simulink model "sampleModel7288_pp_1_1"  (R2018a)
settings: Solver=VariableStepAuto  StartTime=0.0  StopTime=10.0  RelTol=1e-3
undefined symbols (not defined in the file): DiscIntNeverNeededParam, sigbuilder_block
libraries: simulink x497
(part 10 of 10)

== system sampleModel7288_pp_1_1/cfblk310/cfblk17 ==
  cfblk1 : Inport
  cfblk10 : Inport  Port=2
  Action Port : ActionPort  ActionType=else
  cfblk13 : Delay
  cfblk14 : Delay
  cfblk3 : Delay  ShowEnablePort=on
      settings: InputPortMap=u0,e6
  cfblk4 : Delay
  cfblk5 : Delay  ShowEnablePort=on
      settings: InputPortMap=u0,e6
  cfblk6 : DiscreteTransferFcn
  cfblk7 : DiscreteIntegrator  SampleTime=-1  OutDataTypeStr=double  ICPrevOutput=DiscIntNeverNeededParam  ICPrevScaledInput=DiscIntNeverNeededParam
  cfblk8 : simulink/Continuous/PID Controller (2DOF)  Controller=PID  TimeDomain=Discrete-time  SampleTime=-1  IntegratorMethod=Forward Euler  FilterMethod=Forward Euler  Form=Parallel  UseFilter=on  ControllerParametersSource=internal  P=1  I=1  D=0  N=100  b=1  c=1  InitialConditionSource=internal  InitialConditionForIntegrator=0  InitialConditionForFilter=0  ExternalReset=none  LimitOutput=off  UpperSaturationLimit=inf  LowerSaturationLimit=-inf  LinearizeAsGain=off  AntiWindupMode=none  Kb=1  TrackingMode=off  Kt=1  PParamMin=[]  PParamMax=[]  IParamMin=[]  IParamMax=[]  DParamMin=[]  DParamMax=[]  NParamMin=[]  NParamMax=[]  bParamMin=[]  bParamMax=[]  cParamMin=[]  cParamMax=[]  KbParamMin=[]  KbParamMax=[]  KtParamMin=[]  KtParamMax=[]  POutMin=[]  POutMax=[]  IOutMin=[]  IOutMax=[]  DOutMin=[]  DOutMax=[]  NOutMin=[]  NOutMax=[]  bOutMin=[]  bOutMax=[]  cOutMin=[]  cOutMax=[]  KbOutMin=[]  KbOutMax=[]  KtOutMin=[]  KtOutMax=[]  IntegratorOutMin=[]  IntegratorOutMax=[]  FilterOutMin=[]  FilterOutMax=[]  SumOutMin=[]  SumOutMax=[]  Sum1OutMin=[]  Sum1OutMax=[]  Sum2OutMin=[]  Sum2OutMax=[]  Sum3OutMin=[]  Sum3OutMax=[]  SumI1OutMin=[]  SumI1OutMax=[]  SumI2OutMin=[]  SumI2OutMax=[]  SumI3OutMin=[]  SumI3OutMax=[]  SumDOutMin=[]  SumDOutMax=[]  SaturationOutMin=[]  SaturationOutMax=[]  IntegratorContinuousStateAttributes=''  IntegratorStateMustResolveToSignalObject=off  IntegratorRTWStateStorageClass=Auto  FilterContinuousStateAttributes=''  FilterStateMustResolveToSignalObject=off  FilterRTWStateStorageClass=Auto  DifferentiatorICPrevScaledInput=0  DifferentiatorOutMin=[]  DifferentiatorOutMax=[]  FilterDiffOutCoefMin=[]  FilterDiffOutCoefMax=[]  SumDenOutMin=[]  SumDenOutMax=[]  SumNumOutMin=[]  SumNumOutMax=[]  ReciprocalOutMin=[]  ReciprocalOutMax=[]  DivideOutMin=[]  DivideOutMax=[]  TunerSelectOption=Transfer Function Based (PID Tuner App)
  cfblk9 : Delay  DelayLengthSource=Input port
      settings: InputPortMap=u0,p1
  cyemi_{1470..1482} (13 alike) : DataTypeConversion  OutDataTypeStr=double
  cfblk2 : Outport
  cfblk11 : Outport  Port=2
  cfblk12 : Outport  Port=3
  wires:
  cfblk9/1 -> cfblk12/1, cfblk11/1, cyemi_1476/1, cyemi_1479/1
  cfblk5/1 -> cfblk2/1, cyemi_1470/1, cyemi_1471/1
  cyemi_1470/1 -> cfblk13/1
  cyemi_1471/1 -> cfblk14/1
  cyemi_1472/1 -> cfblk3/1
  cfblk6/1 -> cyemi_1472/1
  cyemi_1473/1 -> cfblk3/2
  cfblk1/1 -> cyemi_1473/1
  cyemi_1474/1 -> cfblk4/1
  cfblk3/1 -> cyemi_1474/1
  cyemi_1475/1 -> cfblk5/1
  cfblk8/1 -> cyemi_1475/1
  cyemi_1476/1 -> cfblk5/2
  cyemi_1477/1 -> cfblk6/1
  cfblk10/1 -> cyemi_1477/1
  cyemi_1478/1 -> cfblk7/1
  cfblk4/1 -> cyemi_1478/1
  cyemi_1479/1 -> cfblk8/1
  cyemi_1480/1 -> cfblk8/2
  cfblk14/1 -> cyemi_1480/1
  cyemi_1481/1 -> cfblk9/1
  cfblk13/1 -> cyemi_1481/1
  cyemi_1482/1 -> cfblk9/2
  cfblk7/1 -> cyemi_1482/1

== system sampleModel7288_pp_1_1/cfblk311/cfblk18 ==
  cfblk1 : Inport
  cfblk13 : Inport  Port=2
  cfblk14 : Inport  Port=3
  Action Port : ActionPort  ActionType=then
  cfblk10 : simulink/Discrete/Tapped Delay  vinit=0.0  samptime=-1  NumDelays=1  DelayOrder=Oldest  includeCurrent=off
  cfblk11 : simulink/Discrete/Transfer Fcn Lead or Lag  PoleZ=0.95  ZeroZ=0.75  ICPrevOutput=0.0  ICPrevInput=0.0  DoSatur=off
      settings: SourceProductName=Simulink  SourceProductBaseCode=SL
  cfblk12 : DiscreteZeroPole  Poles=[0 0.5]  Gain=1  SampleTime=-1
  cfblk15 : Delay
  cfblk16 : Delay
  cfblk3 : simulink/Discrete/Transfer Fcn Real Zero  ZeroZ=0.75  ICPrevInput=0.0  DoSatur=off
      settings: SourceProductName=Simulink  SourceProductBaseCode=SL
  cfblk4 : DiscreteTransferFcn
  cfblk5 : simulink/Discrete/Transfer Fcn First Order  PoleZ=0.95  ICPrevOutput=0.0  DoSatur=off
      settings: SourceProductName=Simulink
  cfblk6 : DiscreteIntegrator  SampleTime=-1  OutDataTypeStr=double  ICPrevOutput=DiscIntNeverNeededParam  ICPrevScaledInput=DiscIntNeverNeededParam
  cfblk7 : simulink/Discrete/Transfer Fcn Lead or Lag  PoleZ=0.95  ZeroZ=0.75  ICPrevOutput=0.0  ICPrevInput=0.0  DoSatur=off
      settings: SourceProductName=Simulink  SourceProductBaseCode=SL
  cfblk8 : Delay  ShowEnablePort=on
      settings: InputPortMap=u0,e6
  cfblk9 : simulink/Discrete/Transfer Fcn Real Zero  ZeroZ=0.75  ICPrevInput=0.0  DoSatur=off
      settings: SourceProductName=Simulink  SourceProductBaseCode=SL
  cyemi_{1502..1514} (13 alike) : DataTypeConversion  OutDataTypeStr=double
  cfblk2 : Outport
  wires:
  cfblk5/1 -> cfblk2/1
  cyemi_1502/1 -> cfblk10/1
  cfblk16/1 -> cyemi_1502/1
  cyemi_1503/1 -> cfblk11/1
  cfblk14/1 -> cyemi_1503/1
  cyemi_1504/1 -> cfblk12/1
  cfblk10/1 -> cyemi_1504/1
  cyemi_1505/1 -> cfblk15/1
  cfblk8/1 -> cyemi_1505/1
  cyemi_1506/1 -> cfblk16/1
  cfblk12/1 -> cyemi_1506/1
  cyemi_1507/1 -> cfblk3/1
  cfblk7/1 -> cyemi_1507/1
  cyemi_1508/1 -> cfblk4/1
  cfblk15/1 -> cyemi_1508/1
  cyemi_1509/1 -> cfblk5/1
  cfblk3/1 -> cyemi_1509/1
  cyemi_1510/1 -> cfblk6/1
  cfblk13/1 -> cyemi_1510/1
  cyemi_1511/1 -> cfblk7/1
  cfblk9/1 -> cyemi_1511/1
  cyemi_1512/1 -> cfblk8/1
  cfblk4/1 -> cyemi_1512/1
  cyemi_1513/1 -> cfblk8/2
  cfblk6/1 -> cyemi_1513/1
  cyemi_1514/1 -> cfblk9/1
  cfblk1/1 -> cyemi_1514/1

== system sampleModel7288_pp_1_1/cfblk311/cfblk19 ==
  cfblk1 : Inport
  Action Port : ActionPort  ActionType=else
  cfblk10 : Delay
  cfblk3 : simulink/Discrete/Tapped Delay  vinit=0.0  samptime=-1  NumDelays=1  DelayOrder=Oldest  includeCurrent=off
  cfblk4 : simulink/Discrete/Tapped Delay  vinit=0.0  samptime=-1  NumDelays=1  DelayOrder=Oldest  includeCurrent=off
  cfblk5 : UnitDelay  SampleTime=-1
  cfblk6 : Delay  ShowEnablePort=on
      settings: InputPortMap=u0,e6
  cfblk7 : DiscreteZeroPole  Poles=[0 0.5]  Gain=1  SampleTime=-1
  cfblk9 : Delay
  cyemi_{1516..1519,1521..1523} (7 alike) : DataTypeConversion  OutDataTypeStr=double
  cyemi_1520 : DataTypeConversion  OutDataTypeStr=uint32
  cfblk2 : Outport
  cfblk8 : Outport  Port=2
  wires:
  cfblk6/1 -> cfblk2/1
  cfblk7/1 -> cyemi_1516/1, cyemi_1521/1
  cfblk1/1 -> cfblk8/1, cyemi_1520/1
  cyemi_1516/1 -> cfblk10/1
  cyemi_1517/1 -> cfblk3/1
  cfblk9/1 -> cyemi_1517/1
  cyemi_1518/1 -> cfblk4/1
  cfblk3/1 -> cyemi_1518/1
  cyemi_1519/1 -> cfblk5/1
  cfblk10/1 -> cyemi_1519/1
  cyemi_1520/1 -> cfblk6/1
  cyemi_1521/1 -> cfblk6/2
  cyemi_1522/1 -> cfblk7/1
  cfblk5/1 -> cyemi_1522/1
  cyemi_1523/1 -> cfblk9/1
  cfblk4/1 -> cyemi_1523/1

== system sampleModel7288_pp_1_1/cfblk312/cfblk15 ==
  cfblk1 : Inport
  cfblk16 : Inport  Port=2
  Action Port : ActionPort  ActionType=then
  cfblk10 : simulink/Discrete/Transfer Fcn First Order  PoleZ=0.95  ICPrevOutput=0.0  DoSatur=off
      settings: SourceProductName=Simulink
  cfblk11 : DiscreteIntegrator  SampleTime=-1  OutDataTypeStr=double  ICPrevOutput=DiscIntNeverNeededParam  ICPrevScaledInput=DiscIntNeverNeededParam
  cfblk12 : Delay
  cfblk13 : simulink/Discrete/Difference  ICPrevInput=0.0  OutMin=[]  OutMax=[]  OutDataTypeStr=double  OutputDataTypeScalingMode=double  OutDataType=fixdt(1, 16)  OutScaling=2^-10  DoSatur=off
  cfblk14 : simulink/Continuous/PID Controller (2DOF)  Controller=PID  TimeDomain=Discrete-time  SampleTime=-1  IntegratorMethod=Forward Euler  FilterMethod=Forward Euler  Form=Parallel  UseFilter=on  ControllerParametersSource=internal  P=1  I=1  D=0  N=100  b=1  c=1  InitialConditionSource=internal  InitialConditionForIntegrator=0  InitialConditionForFilter=0  ExternalReset=none  LimitOutput=off  UpperSaturationLimit=inf  LowerSaturationLimit=-inf  LinearizeAsGain=off  AntiWindupMode=none  Kb=1  TrackingMode=off  Kt=1  PParamMin=[]  PParamMax=[]  IParamMin=[]  IParamMax=[]  DParamMin=[]  DParamMax=[]  NParamMin=[]  NParamMax=[]  bParamMin=[]  bParamMax=[]  cParamMin=[]  cParamMax=[]  KbParamMin=[]  KbParamMax=[]  KtParamMin=[]  KtParamMax=[]  POutMin=[]  POutMax=[]  IOutMin=[]  IOutMax=[]  DOutMin=[]  DOutMax=[]  NOutMin=[]  NOutMax=[]  bOutMin=[]  bOutMax=[]  cOutMin=[]  cOutMax=[]  KbOutMin=[]  KbOutMax=[]  KtOutMin=[]  KtOutMax=[]  IntegratorOutMin=[]  IntegratorOutMax=[]  FilterOutMin=[]  FilterOutMax=[]  SumOutMin=[]  SumOutMax=[]  Sum1OutMin=[]  Sum1OutMax=[]  Sum2OutMin=[]  Sum2OutMax=[]  Sum3OutMin=[]  Sum3OutMax=[]  SumI1OutMin=[]  SumI1OutMax=[]  SumI2OutMin=[]  SumI2OutMax=[]  SumI3OutMin=[]  SumI3OutMax=[]  SumDOutMin=[]  SumDOutMax=[]  SaturationOutMin=[]  SaturationOutMax=[]  IntegratorContinuousStateAttributes=''  IntegratorStateMustResolveToSignalObject=off  IntegratorRTWStateStorageClass=Auto  FilterContinuousStateAttributes=''  FilterStateMustResolveToSignalObject=off  FilterRTWStateStorageClass=Auto  DifferentiatorICPrevScaledInput=0  DifferentiatorOutMin=[]  DifferentiatorOutMax=[]  FilterDiffOutCoefMin=[]  FilterDiffOutCoefMax=[]  SumDenOutMin=[]  SumDenOutMax=[]  SumNumOutMin=[]  SumNumOutMax=[]  ReciprocalOutMin=[]  ReciprocalOutMax=[]  DivideOutMin=[]  DivideOutMax=[]  TunerSelectOption=Transfer Function Based (PID Tuner App)
  cfblk15 : simulink/Discrete/Transfer Fcn Lead or Lag  PoleZ=0.95  ZeroZ=0.75  ICPrevOutput=0.0  ICPrevInput=0.0  DoSatur=off
      settings: SourceProductName=Simulink  SourceProductBaseCode=SL
  cfblk3 : simulink/Continuous/PID Controller  Controller=PID  TimeDomain=Discrete-time  SampleTime=-1  IntegratorMethod=Forward Euler  FilterMethod=Forward Euler  Form=Parallel  UseFilter=on  ControllerParametersSource=internal  P=1  I=1  D=0  N=100  InitialConditionSource=internal  InitialConditionForIntegrator=0  InitialConditionForFilter=0  ExternalReset=none  LimitOutput=off  UpperSaturationLimit=inf  LowerSaturationLimit=-inf  LinearizeAsGain=off  AntiWindupMode=none  Kb=1  TrackingMode=off  Kt=1  PParamMin=[]  PParamMax=[]  IParamMin=[]  IParamMax=[]  DParamMin=[]  DParamMax=[]  NParamMin=[]  NParamMax=[]  KbParamMin=[]  KbParamMax=[]  KtParamMin=[]  KtParamMax=[]  POutMin=[]  POutMax=[]  IOutMin=[]  IOutMax=[]  DOutMin=[]  DOutMax=[]  NOutMin=[]  NOutMax=[]  KbOutMin=[]  KbOutMax=[]  KtOutMin=[]  KtOutMax=[]  IntegratorOutMin=[]  IntegratorOutMax=[]  FilterOutMin=[]  FilterOutMax=[]  SumOutMin=[]  SumOutMax=[]  SumI1OutMin=[]  SumI1OutMax=[]  SumI2OutMin=[]  SumI2OutMax=[]  SumI3OutMin=[]  SumI3OutMax=[]  SumDOutMin=[]  SumDOutMax=[]  SaturationOutMin=[]  SaturationOutMax=[]  IntegratorContinuousStateAttributes=''  IntegratorStateMustResolveToSignalObject=off  IntegratorRTWStateStorageClass=Auto  FilterContinuousStateAttributes=''  FilterStateMustResolveToSignalObject=off  FilterRTWStateStorageClass=Auto  DifferentiatorICPrevScaledInput=0  DifferentiatorOutMin=[]  DifferentiatorOutMax=[]  FilterDiffOutCoefMin=[]  FilterDiffOutCoefMax=[]  SumDenOutMin=[]  SumDenOutMax=[]  SumNumOutMin=[]  SumNumOutMax=[]  ReciprocalOutMin=[]  ReciprocalOutMax=[]  DivideOutMin=[]  DivideOutMax=[]  TunerSelectOption=Transfer Function Based (PID Tuner App)
  cfblk4 : simulink/Discrete/Transfer Fcn First Order  PoleZ=0.95  ICPrevOutput=0.0  DoSatur=off
      settings: SourceProductName=Simulink
  cfblk5 : simulink/Discrete/Tapped Delay  vinit=0.0  samptime=-1  NumDelays=1  DelayOrder=Oldest  includeCurrent=off
  cfblk6 : simulink/Discrete/Transfer Fcn Real Zero  ZeroZ=0.75  ICPrevInput=0.0  DoSatur=off
      settings: SourceProductName=Simulink  SourceProductBaseCode=SL
  cfblk7 : UnitDelay  SampleTime=-1
  cfblk8 : DiscreteTransferFcn
  cfblk9 : Delay
  cyemi_{1548..1561} (14 alike) : DataTypeConversion  OutDataTypeStr=double
  cfblk2 : Outport
  cfblk17 : Outport  Port=2
  wires:
  cfblk11/1 -> cfblk17/1, cyemi_1556/1
  cfblk15/1 -> cfblk2/1
  cyemi_1548/1 -> cfblk10/1
  cfblk13/1 -> cyemi_1548/1
  cyemi_1549/1 -> cfblk11/1
  cfblk3/1 -> cyemi_1549/1
  cyemi_1550/1 -> cfblk12/1
  cfblk1/1 -> cyemi_1550/1
  cyemi_1551/1 -> cfblk13/1
  cfblk8/1 -> cyemi_1551/1
  cyemi_1552/1 -> cfblk14/1
  cfblk7/1 -> cyemi_1552/1
  cyemi_1553/1 -> cfblk14/2
  cfblk10/1 -> cyemi_1553/1
  cyemi_1554/1 -> cfblk15/1
  cfblk14/1 -> cyemi_1554/1
  cyemi_1555/1 -> cfblk3/1
  cfblk16/1 -> cyemi_1555/1
  cyemi_1556/1 -> cfblk4/1
  cyemi_1557/1 -> cfblk5/1
  cfblk9/1 -> cyemi_1557/1
  cyemi_1558/1 -> cfblk6/1
  cfblk5/1 -> cyemi_1558/1
  cyemi_1559/1 -> cfblk7/1
  cfblk4/1 -> cyemi_1559/1
  cyemi_1560/1 -> cfblk8/1
  cfblk6/1 -> cyemi_1560/1
  cyemi_1561/1 -> cfblk9/1
  cfblk12/1 -> cyemi_1561/1

== system sampleModel7288_pp_1_1/cfblk312/cfblk16 ==
  cfblk1 : Inport
  Action Port : ActionPort  ActionType=else
  cfblk10 : DiscreteFir
  cfblk11 : simulink/Discrete/Transfer Fcn First Order  PoleZ=0.95  ICPrevOutput=0.0  DoSatur=off
      settings: SourceProductName=Simulink
  cfblk{5,12..14} (4 alike) : simulink/Discrete/Tapped Delay  vinit=0.0  samptime=-1  NumDelays=1  DelayOrder=Oldest  includeCurrent=off
  cfblk15 : DiscreteZeroPole  Poles=[0 0.5]  Gain=1  SampleTime=-1
  cfblk16 : DiscreteStateSpace  SampleTime=-1
  cfblk{3,18..20} (4 alike) : Delay
  cfblk4 : Delay  DelayLengthSource=Input port
      settings: InputPortMap=u0,p1
  cfblk6 : simulink/Discrete/Transfer Fcn First Order  PoleZ=0.95  ICPrevOutput=0.0  DoSatur=off
      settings: SourceProductName=Simulink
  cfblk7 : DiscreteStateSpace  SampleTime=-1
  cfblk8 : DiscreteFir
  cfblk9 : simulink/Discrete/Transfer Fcn Lead or Lag  PoleZ=0.95  ZeroZ=0.75  ICPrevOutput=0.0  ICPrevInput=0.0  DoSatur=off
      settings: SourceProductName=Simulink  SourceProductBaseCode=SL
  cyemi_{1563..1580} (18 alike) : DataTypeConversion  OutDataTypeStr=double
  cfblk2 : Outport
  cfblk17 : Outport  Port=2
  wires:
  cfblk16/1 -> cfblk17/1
  cfblk1/1 -> cyemi_1564/1, cyemi_1569/1
  cfblk6/1 -> cfblk2/1, cyemi_1579/1
  cyemi_1563/1 -> cfblk10/1
  cfblk11/1 -> cyemi_1563/1
  cyemi_1564/1 -> cfblk11/1
  cyemi_1565/1 -> cfblk12/1
  cfblk4/1 -> cyemi_1565/1
  cyemi_1566/1 -> cfblk13/1
  cfblk5/1 -> cyemi_1566/1
  cyemi_1567/1 -> cfblk14/1
  cfblk9/1 -> cyemi_1567/1
  cyemi_1568/1 -> cfblk15/1
  cfblk12/1 -> cyemi_1568/1
  cyemi_1569/1 -> cfblk16/1
  cyemi_1570/1 -> cfblk18/1
  cfblk7/1 -> cyemi_1570/1
  cyemi_1571/1 -> cfblk19/1
  cfblk8/1 -> cyemi_1571/1
  cyemi_1572/1 -> cfblk20/1
  cfblk13/1 -> cyemi_1572/1
  cyemi_1573/1 -> cfblk3/1
  cfblk19/1 -> cyemi_1573/1
  cyemi_1574/1 -> cfblk4/1
  cfblk10/1 -> cyemi_1574/1
  cyemi_1575/1 -> cfblk4/2
  cfblk18/1 -> cyemi_1575/1
  cyemi_1576/1 -> cfblk5/1
  cfblk20/1 -> cyemi_1576/1
  cyemi_1577/1 -> cfblk6/1
  cfblk14/1 -> cyemi_1577/1
  cyemi_1578/1 -> cfblk7/1
  cfblk15/1 -> cyemi_1578/1
  cyemi_1579/1 -> cfblk8/1
  cyemi_1580/1 -> cfblk9/1
  cfblk3/1 -> cyemi_1580/1

== system sampleModel7288_pp_1_1/cfblk313/cfblk14 ==
  cfblk1 : Inport
  Action Port : ActionPort  ActionType=then
  cfblk11 : Delay
  cfblk12 : DataTypeConversion  OutDataTypeStr=double
  cfblk13 : DataTypeConversion  OutDataTypeStr=double
  cfblk14 : DataTypeConversion  OutDataTypeStr=uint32
  cfblk15 : DataTypeConversion  OutDataTypeStr=double
  cfblk3 : Delay  DelayLengthSource=Input port
      settings: InputPortMap=u0,p1
  cfblk4 : simulink/Discrete/Transfer Fcn Real Zero  ZeroZ=0.75  ICPrevInput=0.0  DoSatur=off
      settings: SourceProductName=Simulink  SourceProductBaseCode=SL
  cfblk5 : UnitDelay  SampleTime=-1
  cfblk6 : DiscreteFir
  cfblk7 : UnitDelay  SampleTime=-1
  cfblk8 : DiscreteFir
  cyemi_1598 : DataTypeConversion  OutDataTypeStr=fixdt('ufix64_En32')
  cyemi_{1599,1601..1603,1605..1608} (8 alike) : DataTypeConversion  OutDataTypeStr=double
  cyemi_1600 : DataTypeConversion  OutDataTypeStr=fixdt('ufix64_En32')
  cyemi_1604 : DataTypeConversion  OutDataTypeStr=uint32
  cyemi_1609 : DataTypeConversion  OutDataTypeStr=uint32
  cfblk2 : Outport
  cfblk9 : Outport  Port=2
  cfblk10 : Outport  Port=3
  wires:
  cfblk8/1 -> cfblk2/1, cyemi_1598/1
  cfblk3/1 -> cfblk10/1, cfblk9/1
  cfblk14/1 -> cyemi_1604/1, cyemi_1609/1
  cyemi_1598/1 -> cfblk11/1
  cyemi_1599/1 -> cfblk12/1
  cfblk4/1 -> cyemi_1599/1
  cyemi_1600/1 -> cfblk13/1
  cfblk11/1 -> cyemi_1600/1
  cyemi_1601/1 -> cfblk14/1
  cfblk6/1 -> cyemi_1601/1
  cyemi_1602/1 -> cfblk15/1
  cfblk12/1 -> cyemi_1602/1
  cyemi_1603/1 -> cfblk3/1
  cfblk5/1 -> cyemi_1603/1
  cyemi_1604/1 -> cfblk3/2
  cyemi_1605/1 -> cfblk4/1
  cfblk13/1 -> cyemi_1605/1
  cyemi_1606/1 -> cfblk5/1
  cfblk7/1 -> cyemi_1606/1
  cyemi_1607/1 -> cfblk6/1
  cfblk15/1 -> cyemi_1607/1
  cyemi_1608/1 -> cfblk7/1
  cfblk1/1 -> cyemi_1608/1
  cyemi_1609/1 -> cfblk8/1

== system sampleModel7288_pp_1_1/cfblk313/cfblk15 ==
  cfblk1 : Inport
  cfblk14 : Inport  Port=2
  cfblk15 : Inport  Port=3
  Action Port : ActionPort  ActionType=else
  cfblk10 : UnitDelay  SampleTime=-1
  cfblk11 : UnitDelay  SampleTime=-1
  cfblk12 : simulink/Discrete/Difference  ICPrevInput=0.0  OutMin=[]  OutMax=[]  OutDataTypeStr=double  OutputDataTypeScalingMode=double  OutDataType=fixdt(1, 16)  OutScaling=2^-10  DoSatur=off
  cfblk13 : DiscreteFilter
  cfblk3 : Delay  DelayLengthSource=Input port
      settings: InputPortMap=u0,p1
  cfblk4 : DiscreteFilter
  cfblk5 : DiscreteTransferFcn
  cfblk6 : Delay
  cfblk7 : DiscreteFir
  cfblk8 : UnitDelay  SampleTime=-1
  cfblk9 : DiscreteZeroPole  Poles=[0 0.5]  Gain=1  SampleTime=-1
  cyemi_{1613..1624} (12 alike) : DataTypeConversion  OutDataTypeStr=double
  cfblk2 : Outport
  wires:
  cfblk3/1 -> cfblk2/1
  cyemi_1613/1 -> cfblk10/1
  cfblk7/1 -> cyemi_1613/1
  cyemi_1614/1 -> cfblk11/1
  cfblk5/1 -> cyemi_1614/1
  cyemi_1615/1 -> cfblk12/1
  cfblk11/1 -> cyemi_1615/1
  cyemi_1616/1 -> cfblk13/1
  cfblk10/1 -> cyemi_1616/1
  cyemi_1617/1 -> cfblk3/1
  cfblk15/1 -> cyemi_1617/1
  cyemi_1618/1 -> cfblk3/2
  cfblk14/1 -> cyemi_1618/1
  cyemi_1619/1 -> cfblk4/1
  cfblk1/1 -> cyemi_1619/1
  cyemi_1620/1 -> cfblk5/1
  cfblk6/1 -> cyemi_1620/1
  cyemi_1621/1 -> cfblk6/1
  cfblk13/1 -> cyemi_1621/1
  cyemi_1622/1 -> cfblk7/1
  cfblk8/1 -> cyemi_1622/1
  cyemi_1623/1 -> cfblk8/1
  cfblk9/1 -> cyemi_1623/1
  cyemi_1624/1 -> cfblk9/1
  cfblk4/1 -> cyemi_1624/1

== system sampleModel7288_pp_1_1/cfblk314/cfblk10 ==
  cfblk1 : Inport
  cfblk10 : Inport  Port=2
  cfblk11 : Inport  Port=3
  Action Port : ActionPort  ActionType=then
  cfblk3 : simulink/Discrete/Transfer Fcn Real Zero  ZeroZ=0.75  ICPrevInput=0.0  DoSatur=off
      settings: SourceProductName=Simulink  SourceProductBaseCode=SL
  cfblk4 : Delay  ShowEnablePort=on
      settings: InputPortMap=u0,e6
  cfblk5 : DiscreteZeroPole  Poles=[0 0.5]  Gain=1  SampleTime=-1
  cfblk6 : Delay  ShowEnablePort=on
      settings: InputPortMap=u0,e6
  cfblk7 : simulink/Discrete/Transfer Fcn Real Zero  ZeroZ=0.75  ICPrevInput=0.0  DoSatur=off
      settings: SourceProductName=Simulink  SourceProductBaseCode=SL
  cfblk8 : simulink/Continuous/PID Controller  Controller=PID  TimeDomain=Discrete-time  SampleTime=-1  IntegratorMethod=Forward Euler  FilterMethod=Forward Euler  Form=Parallel  UseFilter=on  ControllerParametersSource=internal  P=1  I=1  D=0  N=100  InitialConditionSource=internal  InitialConditionForIntegrator=0  InitialConditionForFilter=0  ExternalReset=none  LimitOutput=off  UpperSaturationLimit=inf  LowerSaturationLimit=-inf  LinearizeAsGain=off  AntiWindupMode=none  Kb=1  TrackingMode=off  Kt=1  PParamMin=[]  PParamMax=[]  IParamMin=[]  IParamMax=[]  DParamMin=[]  DParamMax=[]  NParamMin=[]  NParamMax=[]  KbParamMin=[]  KbParamMax=[]  KtParamMin=[]  KtParamMax=[]  POutMin=[]  POutMax=[]  IOutMin=[]  IOutMax=[]  DOutMin=[]  DOutMax=[]  NOutMin=[]  NOutMax=[]  KbOutMin=[]  KbOutMax=[]  KtOutMin=[]  KtOutMax=[]  IntegratorOutMin=[]  IntegratorOutMax=[]  FilterOutMin=[]  FilterOutMax=[]  SumOutMin=[]  SumOutMax=[]  SumI1OutMin=[]  SumI1OutMax=[]  SumI2OutMin=[]  SumI2OutMax=[]  SumI3OutMin=[]  SumI3OutMax=[]  SumDOutMin=[]  SumDOutMax=[]  SaturationOutMin=[]  SaturationOutMax=[]  IntegratorContinuousStateAttributes=''  IntegratorStateMustResolveToSignalObject=off  IntegratorRTWStateStorageClass=Auto  FilterContinuousStateAttributes=''  FilterStateMustResolveToSignalObject=off  FilterRTWStateStorageClass=Auto  DifferentiatorICPrevScaledInput=0  DifferentiatorOutMin=[]  DifferentiatorOutMax=[]  FilterDiffOutCoefMin=[]  FilterDiffOutCoefMax=[]  SumDenOutMin=[]  SumDenOutMax=[]  SumNumOutMin=[]  SumNumOutMax=[]  ReciprocalOutMin=[]  ReciprocalOutMax=[]  DivideOutMin=[]  DivideOutMax=[]  TunerSelectOption=Transfer Function Based (PID Tuner App)
  cfblk9 : UnitDelay  SampleTime=-1
  cyemi_{1645..1653} (9 alike) : DataTypeConversion  OutDataTypeStr=double
  cfblk2 : Outport
  wires:
  cfblk6/1 -> cfblk2/1
  cyemi_1645/1 -> cfblk3/1
  cfblk9/1 -> cyemi_1645/1
  cyemi_1646/1 -> cfblk4/1
  cfblk1/1 -> cyemi_1646/1
  cyemi_1647/1 -> cfblk4/2
  cfblk7/1 -> cyemi_1647/1
  cyemi_1648/1 -> cfblk5/1
  cfblk10/1 -> cyemi_1648/1
  cyemi_1649/1 -> cfblk6/1
  cfblk3/1 -> cyemi_1649/1
  cyemi_1650/1 -> cfblk6/2
  cfblk11/1 -> cyemi_1650/1
  cyemi_1651/1 -> cfblk7/1
  cfblk5/1 -> cyemi_1651/1
  cyemi_1652/1 -> cfblk8/1
  cfblk4/1 -> cyemi_1652/1
  cyemi_1653/1 -> cfblk9/1
  cfblk8/1 -> cyemi_1653/1

== system sampleModel7288_pp_1_1/cfblk314/cfblk11 ==
  cfblk1 : Inport
  Action Port : ActionPort  ActionType=else
  cfblk10 : Delay
  cfblk3 : DiscreteFir
  cfblk4 : simulink/Discrete/Tapped Delay  vinit=0.0  samptime=-1  NumDelays=1  DelayOrder=Oldest  includeCurrent=off
  cfblk5 : Delay  ShowEnablePort=on
      settings: InputPortMap=u0,e6
  cfblk6 : DiscreteStateSpace  SampleTime=-1
  cfblk7 : simulink/Discrete/Transfer Fcn Real Zero  ZeroZ=0.75  ICPrevInput=0.0  DoSatur=off
      settings: SourceProductName=Simulink  SourceProductBaseCode=SL
  cfblk8 : simulink/Discrete/Tapped Delay  vinit=0.0  samptime=-1  NumDelays=1  DelayOrder=Oldest  includeCurrent=off
  cyemi_{1655..1662} (8 alike) : DataTypeConversion  OutDataTypeStr=double
  cfblk2 : Outport
  cfblk9 : Outport  Port=2
  wires:
  cfblk3/1 -> cyemi_1660/1, cyemi_1662/1
  cfblk1/1 -> cfblk9/1
  cfblk7/1 -> cfblk2/1, cyemi_1657/1
  cyemi_1655/1 -> cfblk10/1
  cfblk5/1 -> cyemi_1655/1
  cyemi_1656/1 -> cfblk3/1
  cfblk10/1 -> cyemi_1656/1
  cyemi_1657/1 -> cfblk4/1
  cyemi_1658/1 -> cfblk5/1
  cfblk6/1 -> cyemi_1658/1
  cyemi_1659/1 -> cfblk5/2
  cfblk4/1 -> cyemi_1659/1
  cyemi_1660/1 -> cfblk6/1
  cyemi_1661/1 -> cfblk7/1
  cfblk8/1 -> cyemi_1661/1
  cyemi_1662/1 -> cfblk8/1

== system sampleModel7288_pp_1_1/cfblk315/cfblk10 ==
  cfblk1 : Inport
  cfblk12 : Inport  Port=2
  cfblk13 : Inport  Port=3
  Action Port : ActionPort  ActionType=else
  cfblk10 : DiscreteZeroPole  Poles=[0 0.5]  Gain=1  SampleTime=-1
  cfblk11 : Delay  ShowEnablePort=on
      settings: InputPortMap=u0,e6
  cfblk15 : Delay
  cfblk3 : DiscreteTransferFcn
  cfblk4 : simulink/Discrete/Transfer Fcn Lead or Lag  PoleZ=0.95  ZeroZ=0.75  ICPrevOutput=0.0  ICPrevInput=0.0  DoSatur=off
      settings: SourceProductName=Simulink  SourceProductBaseCode=SL
  cfblk5 : simulink/Discrete/Difference  ICPrevInput=0.0  OutMin=[]  OutMax=[]  OutDataTypeStr=double  OutputDataTypeScalingMode=double  OutDataType=fixdt(1, 16)  OutScaling=2^-10  DoSatur=off
  cfblk6 : Delay
  cfblk7 : simulink/Continuous/PID Controller  Controller=PID  TimeDomain=Discrete-time  SampleTime=-1  IntegratorMethod=Forward Euler  FilterMethod=Forward Euler  Form=Parallel  UseFilter=on  ControllerParametersSource=internal  P=1  I=1  D=0  N=100  InitialConditionSource=internal  InitialConditionForIntegrator=0  InitialConditionForFilter=0  ExternalReset=none  LimitOutput=off  UpperSaturationLimit=inf  LowerSaturationLimit=-inf  LinearizeAsGain=off  AntiWindupMode=none  Kb=1  TrackingMode=off  Kt=1  PParamMin=[]  PParamMax=[]  IParamMin=[]  IParamMax=[]  DParamMin=[]  DParamMax=[]  NParamMin=[]  NParamMax=[]  KbParamMin=[]  KbParamMax=[]  KtParamMin=[]  KtParamMax=[]  POutMin=[]  POutMax=[]  IOutMin=[]  IOutMax=[]  DOutMin=[]  DOutMax=[]  NOutMin=[]  NOutMax=[]  KbOutMin=[]  KbOutMax=[]  KtOutMin=[]  KtOutMax=[]  IntegratorOutMin=[]  IntegratorOutMax=[]  FilterOutMin=[]  FilterOutMax=[]  SumOutMin=[]  SumOutMax=[]  SumI1OutMin=[]  SumI1OutMax=[]  SumI2OutMin=[]  SumI2OutMax=[]  SumI3OutMin=[]  SumI3OutMax=[]  SumDOutMin=[]  SumDOutMax=[]  SaturationOutMin=[]  SaturationOutMax=[]  IntegratorContinuousStateAttributes=''  IntegratorStateMustResolveToSignalObject=off  IntegratorRTWStateStorageClass=Auto  FilterContinuousStateAttributes=''  FilterStateMustResolveToSignalObject=off  FilterRTWStateStorageClass=Auto  DifferentiatorICPrevScaledInput=0  DifferentiatorOutMin=[]  DifferentiatorOutMax=[]  FilterDiffOutCoefMin=[]  FilterDiffOutCoefMax=[]  SumDenOutMin=[]  SumDenOutMax=[]  SumNumOutMin=[]  SumNumOutMax=[]  ReciprocalOutMin=[]  ReciprocalOutMax=[]  DivideOutMin=[]  DivideOutMax=[]  TunerSelectOption=Transfer Function Based (PID Tuner App)
  cfblk8 : simulink/Discrete/Transfer Fcn Real Zero  ZeroZ=0.75  ICPrevInput=0.0  DoSatur=off
      settings: SourceProductName=Simulink  SourceProductBaseCode=SL
  cfblk9 : Delay  ShowEnablePort=on
      settings: InputPortMap=u0,e6
  cyemi_{1673..1684} (12 alike) : DataTypeConversion  OutDataTypeStr=double
  cfblk2 : Outport
  cfblk14 : Outport  Port=2
  wires:
  cfblk3/1 -> cfblk14/1
  cfblk8/1 -> cfblk2/1
  cfblk7/1 -> cyemi_1676/1, cyemi_1679/1
  cyemi_1673/1 -> cfblk10/1
  cfblk4/1 -> cyemi_1673/1
  cyemi_1674/1 -> cfblk11/1
  cfblk13/1 -> cyemi_1674/1
  cyemi_1675/1 -> cfblk11/2
  cfblk6/1 -> cyemi_1675/1
  cyemi_1676/1 -> cfblk15/1
  cyemi_1677/1 -> cfblk3/1
  cfblk5/1 -> cyemi_1677/1
  cyemi_1678/1 -> cfblk4/1
  cfblk15/1 -> cyemi_1678/1
  cyemi_1679/1 -> cfblk5/1
  cyemi_1680/1 -> cfblk6/1
  cfblk9/1 -> cyemi_1680/1
  cyemi_1681/1 -> cfblk7/1
  cfblk10/1 -> cyemi_1681/1
  cyemi_1682/1 -> cfblk8/1
  cfblk11/1 -> cyemi_1682/1
  cyemi_1683/1 -> cfblk9/1
  cfblk1/1 -> cyemi_1683/1
  cyemi_1684/1 -> cfblk9/2
  cfblk12/1 -> cyemi_1684/1

== system sampleModel7288_pp_1_1/cfblk315/cfblk9 ==
  cfblk1 : Inport
  Action Port : ActionPort  ActionType=then
  cfblk3 : simulink/Discrete/Difference  ICPrevInput=0.0  OutMin=[]  OutMax=[]  OutDataTypeStr=double  OutputDataTypeScalingMode=double  OutDataType=fixdt(1, 16)  OutScaling=2^-10  DoSatur=off
  cfblk4 : simulink/Continuous/PID Controller  Controller=PID  TimeDomain=Discrete-time  SampleTime=-1  IntegratorMethod=Forward Euler  FilterMethod=Forward Euler  Form=Parallel  UseFilter=on  ControllerParametersSource=internal  P=1  I=1  D=0  N=100  InitialConditionSource=internal  InitialConditionForIntegrator=0  InitialConditionForFilter=0  ExternalReset=none  LimitOutput=off  UpperSaturationLimit=inf  LowerSaturationLimit=-inf  LinearizeAsGain=off  AntiWindupMode=none  Kb=1  TrackingMode=off  Kt=1  PParamMin=[]  PParamMax=[]  IParamMin=[]  IParamMax=[]  DParamMin=[]  DParamMax=[]  NParamMin=[]  NParamMax=[]  KbParamMin=[]  KbParamMax=[]  KtParamMin=[]  KtParamMax=[]  POutMin=[]  POutMax=[]  IOutMin=[]  IOutMax=[]  DOutMin=[]  DOutMax=[]  NOutMin=[]  NOutMax=[]  KbOutMin=[]  KbOutMax=[]  KtOutMin=[]  KtOutMax=[]  IntegratorOutMin=[]  IntegratorOutMax=[]  FilterOutMin=[]  FilterOutMax=[]  SumOutMin=[]  SumOutMax=[]  SumI1OutMin=[]  SumI1OutMax=[]  SumI2OutMin=[]  SumI2OutMax=[]  SumI3OutMin=[]  SumI3OutMax=[]  SumDOutMin=[]  SumDOutMax=[]  SaturationOutMin=[]  SaturationOutMax=[]  IntegratorContinuousStateAttributes=''  IntegratorStateMustResolveToSignalObject=off  IntegratorRTWStateStorageClass=Auto  FilterContinuousStateAttributes=''  FilterStateMustResolveToSignalObject=off  FilterRTWStateStorageClass=Auto  DifferentiatorICPrevScaledInput=0  DifferentiatorOutMin=[]  DifferentiatorOutMax=[]  FilterDiffOutCoefMin=[]  FilterDiffOutCoefMax=[]  SumDenOutMin=[]  SumDenOutMax=[]  SumNumOutMin=[]  SumNumOutMax=[]  ReciprocalOutMin=[]  ReciprocalOutMax=[]  DivideOutMin=[]  DivideOutMax=[]  TunerSelectOption=Transfer Function Based (PID Tuner App)
  cfblk5 : simulink/Continuous/PID Controller  Controller=PID  TimeDomain=Discrete-time  SampleTime=-1  IntegratorMethod=Forward Euler  FilterMethod=Forward Euler  Form=Parallel  UseFilter=on  ControllerParametersSource=internal  P=1  I=1  D=0  N=100  InitialConditionSource=internal  InitialConditionForIntegrator=0  InitialConditionForFilter=0  ExternalReset=none  LimitOutput=off  UpperSaturationLimit=inf  LowerSaturationLimit=-inf  LinearizeAsGain=off  AntiWindupMode=none  Kb=1  TrackingMode=off  Kt=1  PParamMin=[]  PParamMax=[]  IParamMin=[]  IParamMax=[]  DParamMin=[]  DParamMax=[]  NParamMin=[]  NParamMax=[]  KbParamMin=[]  KbParamMax=[]  KtParamMin=[]  KtParamMax=[]  POutMin=[]  POutMax=[]  IOutMin=[]  IOutMax=[]  DOutMin=[]  DOutMax=[]  NOutMin=[]  NOutMax=[]  KbOutMin=[]  KbOutMax=[]  KtOutMin=[]  KtOutMax=[]  IntegratorOutMin=[]  IntegratorOutMax=[]  FilterOutMin=[]  FilterOutMax=[]  SumOutMin=[]  SumOutMax=[]  SumI1OutMin=[]  SumI1OutMax=[]  SumI2OutMin=[]  SumI2OutMax=[]  SumI3OutMin=[]  SumI3OutMax=[]  SumDOutMin=[]  SumDOutMax=[]  SaturationOutMin=[]  SaturationOutMax=[]  IntegratorContinuousStateAttributes=''  IntegratorStateMustResolveToSignalObject=off  IntegratorRTWStateStorageClass=Auto  FilterContinuousStateAttributes=''  FilterStateMustResolveToSignalObject=off  FilterRTWStateStorageClass=Auto  DifferentiatorICPrevScaledInput=0  DifferentiatorOutMin=[]  DifferentiatorOutMax=[]  FilterDiffOutCoefMin=[]  FilterDiffOutCoefMax=[]  SumDenOutMin=[]  SumDenOutMax=[]  SumNumOutMin=[]  SumNumOutMax=[]  ReciprocalOutMin=[]  ReciprocalOutMax=[]  DivideOutMin=[]  DivideOutMax=[]  TunerSelectOption=Transfer Function Based (PID Tuner App)
  cfblk6 : simulink/Discrete/Tapped Delay  vinit=0.0  samptime=-1  NumDelays=1  DelayOrder=Oldest  includeCurrent=off
  cyemi_{1692..1695} (4 alike) : DataTypeConversion  OutDataTypeStr=double
  cfblk2 : Outport
  cfblk7 : Outport  Port=2
  wires:
  cfblk5/1 -> cfblk2/1, cyemi_1695/1
  cfblk3/1 -> cfblk7/1
  cyemi_1692/1 -> cfblk3/1
  cfblk6/1 -> cyemi_1692/1
  cyemi_1693/1 -> cfblk4/1
  cfblk1/1 -> cyemi_1693/1
  cyemi_1694/1 -> cfblk5/1
  cfblk4/1 -> cyemi_1694/1
  cyemi_1695/1 -> cfblk6/1

== system sampleModel7288_pp_1_1/cfblk316/cfblk10 ==
  cfblk1 : Inport
  cfblk15 : Inport  Port=2
  Action Port : ActionPort  ActionType=then
  cfblk10 : DiscreteFir
  cfblk11 : simulink/Continuous/PID Controller (2DOF)  Controller=PID  TimeDomain=Discrete-time  SampleTime=-1  IntegratorMethod=Forward Euler  FilterMethod=Forward Euler  Form=Parallel  UseFilter=on  ControllerParametersSource=internal  P=1  I=1  D=0  N=100  b=1  c=1  InitialConditionSource=internal  InitialConditionForIntegrator=0  InitialConditionForFilter=0  ExternalReset=none  LimitOutput=off  UpperSaturationLimit=inf  LowerSaturationLimit=-inf  LinearizeAsGain=off  AntiWindupMode=none  Kb=1  TrackingMode=off  Kt=1  PParamMin=[]  PParamMax=[]  IParamMin=[]  IParamMax=[]  DParamMin=[]  DParamMax=[]  NParamMin=[]  NParamMax=[]  bParamMin=[]  bParamMax=[]  cParamMin=[]  cParamMax=[]  KbParamMin=[]  KbParamMax=[]  KtParamMin=[]  KtParamMax=[]  POutMin=[]  POutMax=[]  IOutMin=[]  IOutMax=[]  DOutMin=[]  DOutMax=[]  NOutMin=[]  NOutMax=[]  bOutMin=[]  bOutMax=[]  cOutMin=[]  cOutMax=[]  KbOutMin=[]  KbOutMax=[]  KtOutMin=[]  KtOutMax=[]  IntegratorOutMin=[]  IntegratorOutMax=[]  FilterOutMin=[]  FilterOutMax=[]  SumOutMin=[]  SumOutMax=[]  Sum1OutMin=[]  Sum1OutMax=[]  Sum2OutMin=[]  Sum2OutMax=[]  Sum3OutMin=[]  Sum3OutMax=[]  SumI1OutMin=[]  SumI1OutMax=[]  SumI2OutMin=[]  SumI2OutMax=[]  SumI3OutMin=[]  SumI3OutMax=[]  SumDOutMin=[]  SumDOutMax=[]  SaturationOutMin=[]  SaturationOutMax=[]  IntegratorContinuousStateAttributes=''  IntegratorStateMustResolveToSignalObject=off  IntegratorRTWStateStorageClass=Auto  FilterContinuousStateAttributes=''  FilterStateMustResolveToSignalObject=off  FilterRTWStateStorageClass=Auto  DifferentiatorICPrevScaledInput=0  DifferentiatorOutMin=[]  DifferentiatorOutMax=[]  FilterDiffOutCoefMin=[]  FilterDiffOutCoefMax=[]  SumDenOutMin=[]  SumDenOutMax=[]  SumNumOutMin=[]  SumNumOutMax=[]  ReciprocalOutMin=[]  ReciprocalOutMax=[]  DivideOutMin=[]  DivideOutMax=[]  TunerSelectOption=Transfer Function Based (PID Tuner App)
  cfblk12 : simulink/Discrete/Transfer Fcn Real Zero  ZeroZ=0.75  ICPrevInput=0.0  DoSatur=off
      settings: SourceProductName=Simulink  SourceProductBaseCode=SL
  cfblk13 : simulink/Discrete/Difference  ICPrevInput=0.0  OutMin=[]  OutMax=[]  OutDataTypeStr=double  OutputDataTypeScalingMode=double  OutDataType=fixdt(1, 16)  OutScaling=2^-10  DoSatur=off
  cfblk14 : simulink/Discrete/Transfer Fcn First Order  PoleZ=0.95  ICPrevOutput=0.0  DoSatur=off
      settings: SourceProductName=Simulink
  cfblk18 : Delay
  cfblk19 : Delay
  cfblk3 : Delay  DelayLengthSource=Input port
      settings: InputPortMap=u0,p1
  cfblk4 : DiscreteFir
  cfblk5 : simulink/Discrete/Transfer Fcn First Order  PoleZ=0.95  ICPrevOutput=0.0  DoSatur=off
      settings: SourceProductName=Simulink
  cfblk6 : DiscreteTransferFcn
  cfblk7 : UnitDelay  SampleTime=-1
  cfblk8 : Delay  ShowEnablePort=on
      settings: InputPortMap=u0,e6
  cfblk9 : Delay  DelayLengthSource=Input port
      settings: InputPortMap=u0,p1
  cyemi_{1700..1717} (18 alike) : DataTypeConversion  OutDataTypeStr=double
  cfblk2 : Outport
  cfblk16 : Outport  Port=2
  cfblk17 : Outport  Port=3
  wires:
  cfblk12/1 -> cyemi_1701/1, cyemi_1705/1, cyemi_1708/1
  cfblk10/1 -> cyemi_1711/1, cyemi_1715/1
  cfblk3/1 -> cfblk17/1
  cfblk6/1 -> cfblk2/1, cyemi_1706/1
  cfblk13/1 -> cfblk16/1
  cfblk4/1 -> cyemi_1707/1, cyemi_1716/1
  cyemi_1700/1 -> cfblk10/1
  cfblk1/1 -> cyemi_1700/1
  cyemi_1701/1 -> cfblk11/1
  cyemi_1702/1 -> cfblk11/2
  cfblk19/1 -> cyemi_1702/1
  cyemi_1703/1 -> cfblk12/1
  cfblk5/1 -> cyemi_1703/1
  cyemi_1704/1 -> cfblk13/1
  cfblk14/1 -> cyemi_1704/1
  cyemi_1705/1 -> cfblk14/1
  cyemi_1706/1 -> cfblk18/1
  cyemi_1707/1 -> cfblk19/1
  cyemi_1708/1 -> cfblk3/1
  cyemi_1709/1 -> cfblk3/2
  cfblk15/1 -> cyemi_1709/1
  cyemi_1710/1 -> cfblk4/1
  cfblk7/1 -> cyemi_1710/1
  cyemi_1711/1 -> cfblk5/1
  cyemi_1712/1 -> cfblk6/1
  cfblk9/1 -> cyemi_1712/1
  cyemi_1713/1 -> cfblk7/1
  cfblk8/1 -> cyemi_1713/1
  cyemi_1714/1 -> cfblk8/1
  cfblk11/1 -> cyemi_1714/1
  cyemi_1715/1 -> cfblk8/2
  cyemi_1716/1 -> cfblk9/1
  cyemi_1717/1 -> cfblk9/2
  cfblk18/1 -> cyemi_1717/1

== system sampleModel7288_pp_1_1/cfblk316/cfblk11 ==
  cfblk1 : Inport
  Action Port : ActionPort  ActionType=else
  cfblk3 : Delay
  cfblk4 : Delay  ShowEnablePort=on
      settings: InputPortMap=u0,e6
  cfblk5 : DiscreteStateSpace  SampleTime=-1
  cfblk6 : DiscreteIntegrator  SampleTime=-1  OutDataTypeStr=double  ICPrevOutput=DiscIntNeverNeededParam  ICPrevScaledInput=DiscIntNeverNeededParam
  cfblk7 : UnitDelay  SampleTime=-1
  cfblk9 : Delay
  cyemi_{1719..1725} (7 alike) : DataTypeConversion  OutDataTypeStr=double
  cfblk2 : Outport
  cfblk8 : Outport  Port=2
  wires:
  cfblk7/1 -> cfblk8/1
  cfblk1/1 -> cfblk2/1
  cfblk4/1 -> cyemi_1724/1, cyemi_1725/1
  cfblk5/1 -> cyemi_1721/1, cyemi_1723/1
  cyemi_1719/1 -> cfblk3/1
  cfblk9/1 -> cyemi_1719/1
  cyemi_1720/1 -> cfblk4/1
  cfblk6/1 -> cyemi_1720/1
  cyemi_1721/1 -> cfblk4/2
  cyemi_1722/1 -> cfblk5/1
  cfblk3/1 -> cyemi_1722/1
  cyemi_1723/1 -> cfblk6/1
  cyemi_1724/1 -> cfblk7/1
  cyemi_1725/1 -> cfblk9/1

== system sampleModel7288_pp_1_1/cfblk317/cfblk18 ==
  cfblk1 : Inport
  Action Port : ActionPort  ActionType=then
  cfblk10 : simulink/Discrete/Difference  ICPrevInput=0.0  OutMin=[]  OutMax=[]  OutDataTypeStr=double  OutputDataTypeScalingMode=double  OutDataType=fixdt(1, 16)  OutScaling=2^-10  DoSatur=off
  cfblk12 : Delay
  cfblk3 : simulink/Discrete/Difference  ICPrevInput=0.0  OutMin=[]  OutMax=[]  OutDataTypeStr=double  OutputDataTypeScalingMode=double  OutDataType=fixdt(1, 16)  OutScaling=2^-10  DoSatur=off
  cfblk4 : Delay
  cfblk5 : Delay
  cfblk6 : DiscreteZeroPole  Poles=[0 0.5]  Gain=1  SampleTime=-1
  cfblk7 : DiscreteZeroPole  Poles=[0 0.5]  Gain=1  SampleTime=-1
  cfblk8 : simulink/Discrete/Transfer Fcn Real Zero  ZeroZ=0.75  ICPrevInput=0.0  DoSatur=off
      settings: SourceProductName=Simulink  SourceProductBaseCode=SL
  cfblk9 : DiscreteStateSpace  SampleTime=-1
  cyemi_{1742..1750} (9 alike) : DataTypeConversion  OutDataTypeStr=double
  cfblk2 : Outport
  cfblk11 : Outport  Port=2
  wires:
  cfblk10/1 -> cfblk2/1, cyemi_1748/1
  cfblk8/1 -> cfblk11/1
  cyemi_1742/1 -> cfblk10/1
  cfblk3/1 -> cyemi_1742/1
  cyemi_1743/1 -> cfblk12/1
  cfblk9/1 -> cyemi_1743/1
  cyemi_1744/1 -> cfblk3/1
  cfblk5/1 -> cyemi_1744/1
  cyemi_1745/1 -> cfblk4/1
  cfblk12/1 -> cyemi_1745/1
  cyemi_1746/1 -> cfblk5/1
  cfblk1/1 -> cyemi_1746/1
  cyemi_1747/1 -> cfblk6/1
  cfblk4/1 -> cyemi_1747/1
  cyemi_1748/1 -> cfblk7/1
  cyemi_1749/1 -> cfblk8/1
  cfblk7/1 -> cyemi_1749/1
  cyemi_1750/1 -> cfblk9/1
  cfblk6/1 -> cyemi_1750/1

== system sampleModel7288_pp_1_1/cfblk317/cfblk19 ==
  cfblk1 : Inport
  cfblk7 : Inport  Port=2
  Action Port : ActionPort  ActionType=else
  cfblk3 : DiscreteTransferFcn
  cfblk4 : simulink/Discrete/Transfer Fcn First Order  PoleZ=0.95  ICPrevOutput=0.0  DoSatur=off
      settings: SourceProductName=Simulink
  cfblk5 : DiscreteZeroPole  Poles=[0 0.5]  Gain=1  SampleTime=-1
  cfblk6 : DiscreteStateSpace  SampleTime=-1
  cyemi_{1753..1756} (4 alike) : DataTypeConversion  OutDataTypeStr=double
  cfblk2 : Outport
  cfblk8 : Outport  Port=2
  wires:
  cfblk4/1 -> cfblk2/1
  cfblk1/1 -> cfblk8/1
  cyemi_1753/1 -> cfblk3/1
  cfblk5/1 -> cyemi_1753/1
  cyemi_1754/1 -> cfblk4/1
  cfblk3/1 -> cyemi_1754/1
  cyemi_1755/1 -> cfblk5/1
  cfblk6/1 -> cyemi_1755/1
  cyemi_1756/1 -> cfblk6/1
  cfblk7/1 -> cyemi_1756/1

== system sampleModel7288_pp_1_1/cfblk318/cfblk16 ==
  cfblk1 : Inport
  cfblk15 : Inport  Port=2
  Action Port : ActionPort  ActionType=then
  cfblk10 : simulink/Discrete/Transfer Fcn Lead or Lag  PoleZ=0.95  ZeroZ=0.75  ICPrevOutput=0.0  ICPrevInput=0.0  DoSatur=off
      settings: SourceProductName=Simulink  SourceProductBaseCode=SL
  cfblk11 : simulink/Discrete/Tapped Delay  vinit=0.0  samptime=-1  NumDelays=1  DelayOrder=Oldest  includeCurrent=off
  cfblk12 : DiscreteFilter
  cfblk13 : simulink/Discrete/Transfer Fcn Real Zero  ZeroZ=0.75  ICPrevInput=0.0  DoSatur=off
      settings: SourceProductName=Simulink  SourceProductBaseCode=SL
  cfblk14 : Delay  ShowEnablePort=on
      settings: InputPortMap=u0,e6
  cfblk16 : Delay
  cfblk3 : simulink/Discrete/Tapped Delay  vinit=0.0  samptime=-1  NumDelays=1  DelayOrder=Oldest  includeCurrent=off
  cfblk4 : UnitDelay  SampleTime=-1
  cfblk5 : DiscreteFilter
  cfblk6 : DiscreteZeroPole  Poles=[0 0.5]  Gain=1  SampleTime=-1
  cfblk7 : DiscreteStateSpace  SampleTime=-1
  cfblk8 : DiscreteFilter
  cfblk9 : DiscreteFir
  cyemi_{1775..1788} (14 alike) : DataTypeConversion  OutDataTypeStr=double
  cfblk2 : Outport
  wires:
  cfblk4/1 -> cfblk2/1
  cfblk14/1 -> cyemi_1778/1, cyemi_1782/1
  cyemi_1775/1 -> cfblk10/1
  cfblk15/1 -> cyemi_1775/1
  cyemi_1776/1 -> cfblk11/1
  cfblk6/1 -> cyemi_1776/1
  cyemi_1777/1 -> cfblk12/1
  cfblk9/1 -> cyemi_1777/1
  cyemi_1778/1 -> cfblk13/1
  cyemi_1779/1 -> cfblk14/1
  cfblk16/1 -> cyemi_1779/1
  cyemi_1780/1 -> cfblk14/2
  cfblk8/1 -> cyemi_1780/1
  cyemi_1781/1 -> cfblk16/1
  cfblk12/1 -> cyemi_1781/1
  cyemi_1782/1 -> cfblk3/1
  cyemi_1783/1 -> cfblk4/1
  cfblk11/1 -> cyemi_1783/1
  cyemi_1784/1 -> cfblk5/1
  cfblk10/1 -> cyemi_1784/1
  cyemi_1785/1 -> cfblk6/1
  cfblk7/1 -> cyemi_1785/1
  cyemi_1786/1 -> cfblk7/1
  cfblk5/1 -> cyemi_1786/1
  cyemi_1787/1 -> cfblk8/1
  cfblk1/1 -> cyemi_1787/1
  cyemi_1788/1 -> cfblk9/1
  cfblk3/1 -> cyemi_1788/1

== system sampleModel7288_pp_1_1/cfblk318/cfblk17 ==
  cfblk1 : Inport
  cfblk13 : Inport  Port=2
  cfblk14 : Inport  Port=3
  cfblk15 : Inport  Port=4
  Action Port : ActionPort  ActionType=else
  cfblk10 : simulink/Discrete/Transfer Fcn Real Zero  ZeroZ=0.75  ICPrevInput=0.0  DoSatur=off
      settings: SourceProductName=Simulink  SourceProductBaseCode=SL
  cfblk11 : simulink/Discrete/Transfer Fcn Lead or Lag  PoleZ=0.95  ZeroZ=0.75  ICPrevOutput=0.0  ICPrevInput=0.0  DoSatur=off
      settings: SourceProductName=Simulink  SourceProductBaseCode=SL
  cfblk12 : DiscreteIntegrator  SampleTime=-1  OutDataTypeStr=double  ICPrevOutput=DiscIntNeverNeededParam  ICPrevScaledInput=DiscIntNeverNeededParam
  cfblk3 : DiscreteIntegrator  SampleTime=-1  OutDataTypeStr=double  ICPrevOutput=DiscIntNeverNeededParam  ICPrevScaledInput=DiscIntNeverNeededParam
  cfblk4 : UnitDelay  SampleTime=-1
  cfblk5 : DiscreteFir
  cfblk6 : simulink/Discrete/Transfer Fcn First Order  PoleZ=0.95  ICPrevOutput=0.0  DoSatur=off
      settings: SourceProductName=Simulink
  cfblk7 : DiscreteFilter
  cfblk8 : DiscreteFilter
  cfblk9 : simulink/Continuous/PID Controller  Controller=PID  TimeDomain=Discrete-time  SampleTime=-1  IntegratorMethod=Forward Euler  FilterMethod=Forward Euler  Form=Parallel  UseFilter=on  ControllerParametersSource=internal  P=1  I=1  D=0  N=100  InitialConditionSource=internal  InitialConditionForIntegrator=0  InitialConditionForFilter=0  ExternalReset=none  LimitOutput=off  UpperSaturationLimit=inf  LowerSaturationLimit=-inf  LinearizeAsGain=off  AntiWindupMode=none  Kb=1  TrackingMode=off  Kt=1  PParamMin=[]  PParamMax=[]  IParamMin=[]  IParamMax=[]  DParamMin=[]  DParamMax=[]  NParamMin=[]  NParamMax=[]  KbParamMin=[]  KbParamMax=[]  KtParamMin=[]  KtParamMax=[]  POutMin=[]  POutMax=[]  IOutMin=[]  IOutMax=[]  DOutMin=[]  DOutMax=[]  NOutMin=[]  NOutMax=[]  KbOutMin=[]  KbOutMax=[]  KtOutMin=[]  KtOutMax=[]  IntegratorOutMin=[]  IntegratorOutMax=[]  FilterOutMin=[]  FilterOutMax=[]  SumOutMin=[]  SumOutMax=[]  SumI1OutMin=[]  SumI1OutMax=[]  SumI2OutMin=[]  SumI2OutMax=[]  SumI3OutMin=[]  SumI3OutMax=[]  SumDOutMin=[]  SumDOutMax=[]  SaturationOutMin=[]  SaturationOutMax=[]  IntegratorContinuousStateAttributes=''  IntegratorStateMustResolveToSignalObject=off  IntegratorRTWStateStorageClass=Auto  FilterContinuousStateAttributes=''  FilterStateMustResolveToSignalObject=off  FilterRTWStateStorageClass=Auto  DifferentiatorICPrevScaledInput=0  DifferentiatorOutMin=[]  DifferentiatorOutMax=[]  FilterDiffOutCoefMin=[]  FilterDiffOutCoefMax=[]  SumDenOutMin=[]  SumDenOutMax=[]  SumNumOutMin=[]  SumNumOutMax=[]  ReciprocalOutMin=[]  ReciprocalOutMax=[]  DivideOutMin=[]  DivideOutMax=[]  TunerSelectOption=Transfer Function Based (PID Tuner App)
  cyemi_{1793..1802} (10 alike) : DataTypeConversion  OutDataTypeStr=double
  cfblk2 : Outport
  wires:
  cfblk7/1 -> cfblk2/1
  cyemi_1793/1 -> cfblk10/1
  cfblk8/1 -> cyemi_1793/1
  cyemi_1794/1 -> cfblk11/1
  cfblk9/1 -> cyemi_1794/1
  cyemi_1795/1 -> cfblk12/1
  cfblk15/1 -> cyemi_1795/1
  cyemi_1796/1 -> cfblk3/1
  cfblk14/1 -> cyemi_1796/1
  cyemi_1797/1 -> cfblk4/1
  cfblk10/1 -> cyemi_1797/1
  cyemi_1798/1 -> cfblk5/1
  cfblk12/1 -> cyemi_1798/1
  cyemi_1799/1 -> cfblk6/1
  cfblk13/1 -> cyemi_1799/1
  cyemi_1800/1 -> cfblk7/1
  cfblk11/1 -> cyemi_1800/1
  cyemi_1801/1 -> cfblk8/1
  cfblk3/1 -> cyemi_1801/1
  cyemi_1802/1 -> cfblk9/1
  cfblk1/1 -> cyemi_1802/1
